simulink model "TV_lisb"  (R2024b)
settings: Solver=VariableStepAuto  StartTime=0.0  StopTime=10.0  RelTol=1e-3
PreLoadFcn:
  | run("TV_lisb_helper_file.m")
PostLoadFcn:
  | run("TV_lisb_helper_file.m")
InitFcn:
  | run("TV_lisb_helper_file.m")
StartFcn:
  | run("TV_lisb_helper_file.m")
StopFcn:
  | run("TV_lisb_helper_file.m")
model workspace: external: MATLAB File C:\Users\USER\Documents\MATLAB\NR\Git\TV_lisb_helper_file.m (data not in the file)
values from neighbouring files (symbols this model uses):
  C1 = 1.28    [TV_lisb_helper_file.m]
  C2 = 23.99    [TV_lisb_helper_file.m]
  C3 = 0.52    [TV_lisb_helper_file.m]
  C_roll = 0.01    [TV_lisb_helper_file.m]
  lf = 1.5    [TV_lisb_helper_file.m]
  lr = 1.5    [TV_lisb_helper_file.m]
  M = 300    [TV_lisb_helper_file.m]
  wr = 0.22    [TV_lisb_helper_file.m]
undefined symbols (not defined in the file or in its folder): g, tr
libraries: simulink x1
PreSaveFcn:
  | run("TV_lisb_helper_file.m")
PostSaveFcn:
  | run("TV_lisb_helper_file.m")
CloseFcn:
  | run("TV_lisb_helper_file.m")
PauseFcn:
  | run("TV_lisb_helper_file.m")
ContinueFcn:
  | run("TV_lisb_helper_file.m")
settings Model: Creator=USER  LastModifiedBy=USER

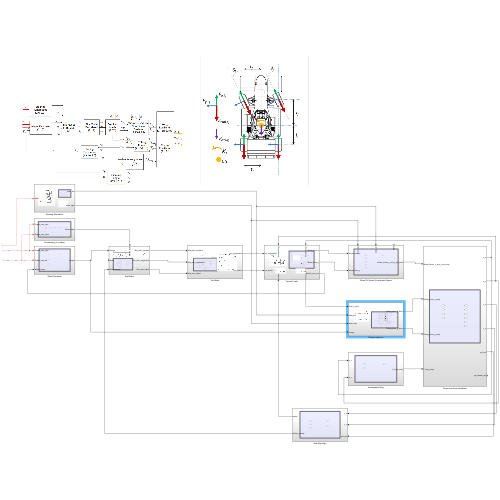
[thumbnail: Simulink's stored preview of the top-level diagram]
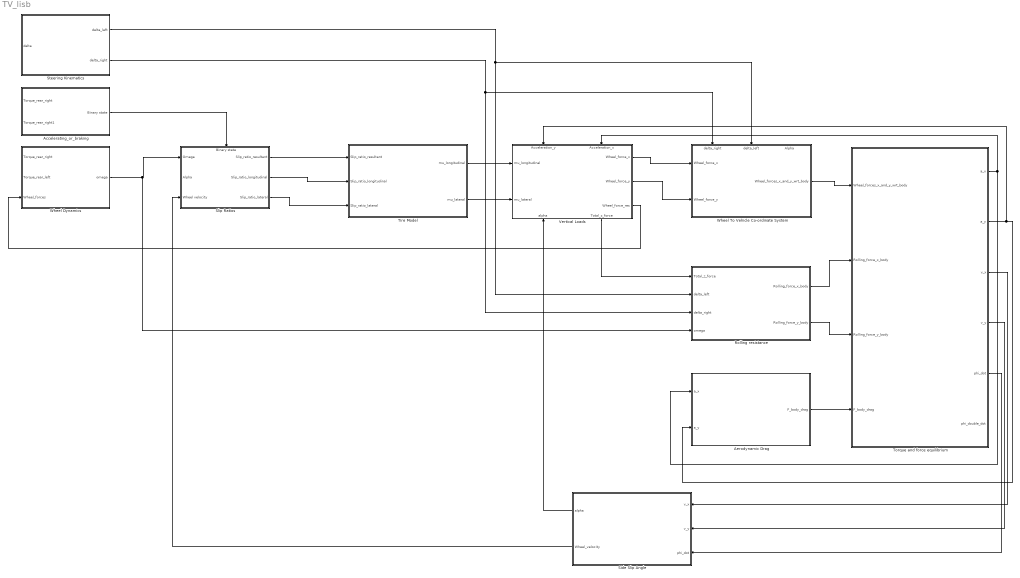
== system TV_lisb ==
  Accelerating_or_braking : Subsystem
  Aerodynamic Drag : Subsystem
  Rolling resistance : Subsystem
  Side Slip Angle : Subsystem
  Slip Ratios : Subsystem
      settings: PortSchema="{\"entries\":[{\"content\":{\"sides\":[{\"content\":{\"connectorIds\":[\"In1\",\"In2\",\"In3\"]},\"type\":\"ConnectorPlacement.EquallySpacedRectSide\",\"uuid\":\"f68f1183-9c60-479b-925c-3d4ffcaa1183\"},{\"content\":{\"connectorIds\":[\"Out1\",\"Out2\",\"Out3\"],\"side\":\"RIGHT\"},\"type\":\"ConnectorPlacement.EquallySpacedRectSide\",\"uuid\":\"3ccc78e5-55f6-4f64-bd15-35f9b9c5843d\"},{\"content\":{\"connectorIds\":[\"In4\"],\"side\":\"TOP\"},\"type\":\"ConnectorPlacement.EquallySpacedRectSide\",\"uuid\":\"873faff7-faeb-472b-bbf0-059c7e3a1cec\"}]},\"type\":\"ConnectorPlacement.EquallySpacedConnector\",\"uuid\":\"c1430164-14ee-465b-ad5a-b929bb7f1d2a\"}],\"packageUris\":[\"http://schema.mathworks.com/mf0/Connector/R2020b\"],\"version\":\"1.0\"}"
  Steering Kinematics : Subsystem
  Tire Model : Subsystem
  Torque and force equilibrium : Subsystem
  Vertical Loads : Subsystem
      settings: PortSchema="{\"entries\":[{\"content\":{\"sides\":[{\"content\":{\"connectorIds\":[\"In1\",\"In2\"]},\"type\":\"ConnectorPlacement.EquallySpacedRectSide\",\"uuid\":\"420474dd-77ae-41a3-b184-b8a376845dee\"},{\"content\":{\"connectorIds\":[\"Out1\",\"Out2\",\"Out3\"],\"side\":\"RIGHT\"},\"type\":\"ConnectorPlacement.EquallySpacedRectSide\",\"uuid\":\"e98bfd49-6816-4384-b726-feedfd108428\"},{\"content\":{\"connectorIds\":[\"In3\",\"In4\"],\"side\":\"TOP\"},\"type\":\"ConnectorPlacement.EquallySpacedRectSide\",\"uuid\":\"bc3c4692-54cb-49d4-bb5f-a504cda1efb8\"},{\"content\":{\"connectorIds\":[\"In5\",\"Out4\"],\"side\":\"BOTTOM\"},\"type\":\"ConnectorPlacement.EquallySpacedRectSide\",\"uuid\":\"ec39efe8-9589-4d25-8c83-c5c7b2f70cfd\"}]},\"type\":\"ConnectorPlacement.EquallySpacedConnector\",\"uuid\":\"6b01247e-c69a-46fe-b6d9-037bfd45934f\"}],\"packageUris\":[\"http://schema.mathworks.com/mf0/Connector/R2020b\"],\"version\":\"1.0\"}"
  Wheel Dynamics : Subsystem
  Wheel To Vehicle Co-ordinate System : Subsystem
      settings: PortSchema="{\"entries\":[{\"content\":{\"sides\":[{\"content\":{\"connectorIds\":[\"In1\",\"In2\"]},\"type\":\"ConnectorPlacement.EquallySpacedRectSide\",\"uuid\":\"1d639fc9-362c-4114-a9a5-2cccb0aa4f8f\"},{\"content\":{\"connectorIds\":[\"Out1\"],\"side\":\"RIGHT\"},\"type\":\"ConnectorPlacement.EquallySpacedRectSide\",\"uuid\":\"af7b8bc1-4639-4e57-ae25-0425d451201b\"},{\"content\":{\"connectorIds\":[\"In3\",\"In4\",\"In5\"],\"side\":\"TOP\"},\"type\":\"ConnectorPlacement.EquallySpacedRectSide\",\"uuid\":\"e7928f69-bff2-45cc-8c36-948ca369821c\"}]},\"type\":\"ConnectorPlacement.EquallySpacedConnector\",\"uuid\":\"c77d5f9f-6196-466d-893b-8bb143925d68\"}],\"packageUris\":[\"http://schema.mathworks.com/mf0/Connector/R2020b\"],\"version\":\"1.0\"}"
  wires:
  Slip Ratios/1(Slip_ratio_resultant) -> Tire Model/1(Slip_ratio_resultant)
  Wheel Dynamics/1(omega) -> Rolling resistance/4(omega), Slip Ratios/1(Omega)
  Vertical Loads/1(Wheel_force_x) -> Wheel To Vehicle Co-ordinate System/1(Wheel_force_x)
  Vertical Loads/2(Wheel_force_y) -> Wheel To Vehicle Co-ordinate System/2(Wheel_force_y)
  Steering Kinematics/2(delta_right) -> Rolling resistance/3(delta_right), Wheel To Vehicle Co-ordinate System/3(delta_right)
  Steering Kinematics/1(delta_left) -> Rolling resistance/2(delta_left), Wheel To Vehicle Co-ordinate System/4(delta_left)
  Wheel To Vehicle Co-ordinate System/1(Wheel_forces_x_and_y_wrt_body) -> Torque and force equilibrium/1(Wheel_forces_x_and_y_wrt_body)
  Vertical Loads/4(Total_z_force) -> Rolling resistance/1(Total_z_force)
  Rolling resistance/1(Rolling_force_x_body) -> Torque and force equilibrium/2(Rolling_force_x_body)
  Rolling resistance/2(Rolling_force_y_body) -> Torque and force equilibrium/3(Rolling_force_y_body)
  Aerodynamic Drag/1(F_body_drag) -> Torque and force equilibrium/4(F_body_drag)
  Torque and force equilibrium/1(a_x) -> Vertical Loads/4(Acceleration_x), Aerodynamic Drag/1(a_x)
  Torque and force equilibrium/2(a_y) -> Aerodynamic Drag/2(a_y), Vertical Loads/3(Acceleration_y)
  Vertical Loads/3(Wheel_force_res) -> Wheel Dynamics/3(Wheel_forces)
  Side Slip Angle/1(alpha) -> Vertical Loads/5(alpha)
  Side Slip Angle/2(Wheel_velocity) -> Slip Ratios/3(Wheel velocity)
  Torque and force equilibrium/3(v_x) -> Side Slip Angle/1(v_x)
  Torque and force equilibrium/4(v_y) -> Side Slip Angle/2(v_y)
  Torque and force equilibrium/5(phi_dot) -> Side Slip Angle/3(phi_dot)
  ? -> Accelerating_or_braking/1(Torque_rear_right), Wheel Dynamics/1(Torque_rear_right)
  ? -> Accelerating_or_braking/2(Torque_rear_right1), Wheel Dynamics/2(Torque_rear_left)
  Accelerating_or_braking/1(Binary state) -> Slip Ratios/4(Binary state)
  ? -> Steering Kinematics/1(delta)
  Slip Ratios/2(Slip_ratio_longitudinal) -> Tire Model/2(Slip_ratio_longitudinal)
  Slip Ratios/3(Slip_ratio_lateral) -> Tire Model/3(Slip_ratio_lateral)
  Tire Model/1(mu_longitudinal) -> Vertical Loads/1(mu_longitudinal)
  Tire Model/2(mu_lateral) -> Vertical Loads/2(mu_lateral)

== system TV_lisb/Accelerating_or_braking ==
  note: Gives 0 for braking, and 1 for accelerating
  Torque_rear_right : Inport
  Torque_rear_right1 : Inport  Port=2
  Add : Sum
  Compare To Zero : simulink/Logic and Bit Operations/Compare To Zero  relop=>=  OutDataTypeStr=uint8
  Derivative : Derivative
  Gain : Gain  Gain=0.5
  Binary state : Outport
  wires:
  Torque_rear_right/1 -> Add/1
  Torque_rear_right1/1 -> Add/2
  Add/1 -> Gain/1
  Gain/1 -> Derivative/1
  Derivative/1 -> Compare To Zero/1
  Compare To Zero/1 -> Binary state/1

== system TV_lisb/Aerodynamic Drag ==
  note: Aero calcs
  a_x : Inport
  a_y : Inport  Port=2
  F_body_drag : Outport

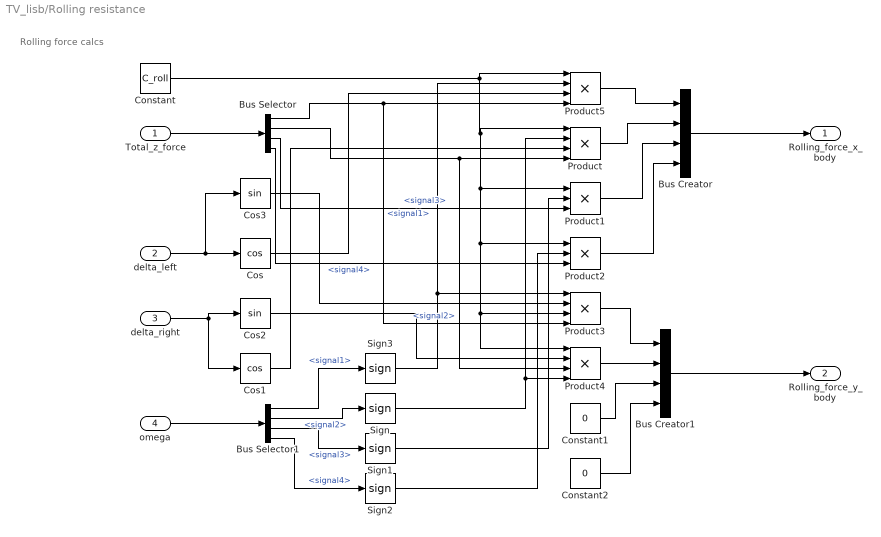
== system TV_lisb/Rolling resistance ==
  note: Rolling force calcs
  Total_z_force : Inport
  delta_left : Inport  Port=2
  delta_right : Inport  Port=3
  omega : Inport  Port=4
  Bus Creator : BusCreator  Inputs=4
  Bus Creator1 : BusCreator  Inputs=4
  Bus Selector : BusSelector  OutputSignals=signal1,signal2,signal3,signal4
  Bus Selector1 : BusSelector  OutputSignals=signal1,signal2,signal3,signal4
  Constant : Constant  Value=C_roll
  Constant1 : Constant  Value=0
  Constant2 : Constant  Value=0
  Cos : Trigonometry  Operator=cos
  Cos1 : Trigonometry  Operator=cos
  Cos2 : Trigonometry
  Cos3 : Trigonometry
  Product{,3..5} (4 alike) : Product  Inputs=4
  Product1 : Product  Inputs=3
  Product2 : Product  Inputs=3
  Sign{,1..3} (4 alike) : Signum
  Rolling_force_x_body : Outport
  Rolling_force_y_body : Outport  Port=2
  wires:
  Total_z_force/1 -> Bus Selector/1
  omega/1 -> Bus Selector1/1
  delta_left/1 -> Cos3/1, Cos/1
  delta_right/1 -> Cos2/1, Cos1/1
  Bus Selector1/1 -> Sign3/1  "<signal1>"
  Bus Selector1/2 -> Sign/1  "<signal2>"
  Bus Selector1/3 -> Sign1/1  "<signal3>"
  Bus Selector1/4 -> Sign2/1  "<signal4>"
  Constant/1 -> Product4/1, Product3/3, Product2/1, Product1/1, Product/1, Product5/1
  Bus Selector/1 -> Product3/4, Product5/4  "<signal1>"
  Sign3/1 -> Product3/1, Product5/2
  Cos/1 -> Product5/3
  Bus Selector/2 -> Product4/3, Product/4  "<signal2>"
  Sign/1 -> Product/2, Product4/4
  Cos1/1 -> Product/3
  Bus Selector/3 -> Product1/3  "<signal3>"
  Bus Selector/4 -> Product2/3  "<signal4>"
  Sign1/1 -> Product1/2
  Sign2/1 -> Product2/2
  Bus Creator/1 -> Rolling_force_x_body/1
  Product5/1 -> Bus Creator/1
  Product/1 -> Bus Creator/2
  Product1/1 -> Bus Creator/3
  Product2/1 -> Bus Creator/4
  Bus Creator1/1 -> Rolling_force_y_body/1
  Constant2/1 -> Bus Creator1/4
  Constant1/1 -> Bus Creator1/3
  Product4/1 -> Bus Creator1/2
  Product3/1 -> Bus Creator1/1
  Cos3/1 -> Product3/2
  Cos2/1 -> Product4/2

== system TV_lisb/Side Slip Angle ==
  note: Slip angle calcs
  v_x : Inport
  v_y : Inport  Port=2
  phi_dot : Inport  Port=3
  alpha : Outport
  Wheel_velocity : Outport  Port=2

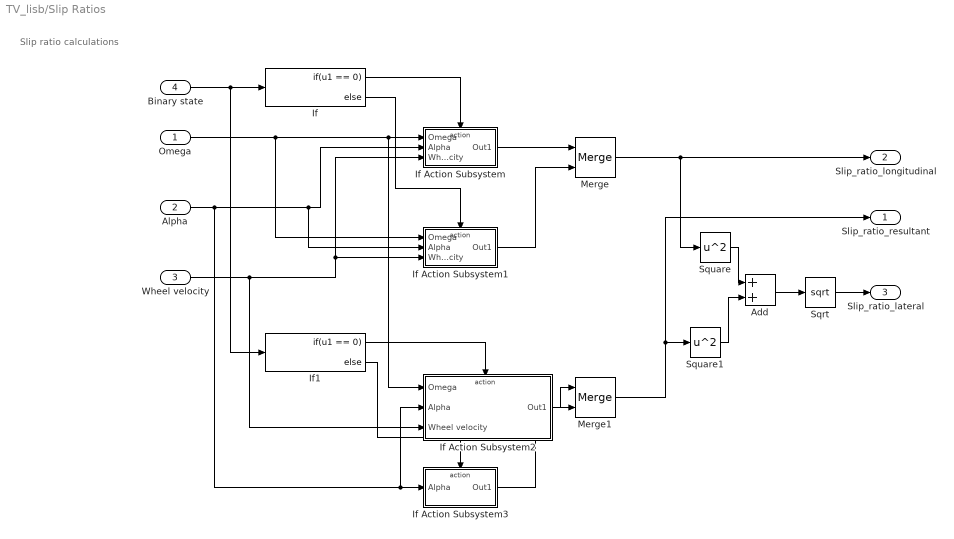
== system TV_lisb/Slip Ratios ==
  note: Slip ratio calculations
  Omega : Inport
  Alpha : Inport  Port=2
  Wheel velocity : Inport  Port=3
  Binary state : Inport  Port=4
  Add : Sum
  If : If  IfExpression=u1 == 0
  If Action Subsystem : Subsystem  TreatAsAtomicUnit=on
  If Action Subsystem1 : Subsystem  TreatAsAtomicUnit=on
  If Action Subsystem2 : Subsystem  TreatAsAtomicUnit=on
  If Action Subsystem3 : Subsystem  TreatAsAtomicUnit=on
  If1 : If  IfExpression=u1 == 0
  Merge : Merge
  Merge1 : Merge
  Sqrt : Sqrt
  Square : Math  Operator=square
  Square1 : Math  Operator=square
  Slip_ratio_resultant : Outport
  Slip_ratio_longitudinal : Outport  Port=2
  Slip_ratio_lateral : Outport  Port=3
  wires:
  Binary state/1 -> If/1, If1/1
  If/1 -> If Action Subsystem/Action
  If/2 -> If Action Subsystem1/Action
  Omega/1 -> If Action Subsystem2/1(Omega), If Action Subsystem/1(Omega), If Action Subsystem1/1(Omega)
  Alpha/1 -> If Action Subsystem1/2(Alpha), If Action Subsystem/2(Alpha), If Action Subsystem2/2(Alpha), If Action Subsystem3/1(Alpha)
  Wheel velocity/1 -> If Action Subsystem2/3(Wheel velocity), If Action Subsystem1/3(Wheel velocity), If Action Subsystem/3(Wheel velocity)
  If Action Subsystem/1(Out1) -> Merge/1
  If Action Subsystem1/1(Out1) -> Merge/2
  Merge/1 -> Square/1, Slip_ratio_longitudinal/1
  If Action Subsystem2/1(Out1) -> Merge1/1
  If Action Subsystem3/1(Out1) -> Merge1/2
  Merge1/1 -> Square1/1, Slip_ratio_resultant/1
  If1/1 -> If Action Subsystem2/Action
  If1/2 -> If Action Subsystem3/Action
  Sqrt/1 -> Slip_ratio_lateral/1
  Add/1 -> Sqrt/1
  Square/1 -> Add/1
  Square1/1 -> Add/2

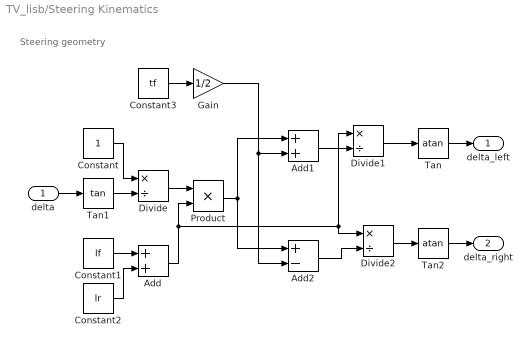
== system TV_lisb/Steering Kinematics ==
  note: Steering geometry
  delta : Inport
  Add : Sum
  Add1 : Sum
  Add2 : Sum  Inputs=+-
  Constant : Constant
  Constant1 : Constant  Value=lf
  Constant2 : Constant  Value=lr
  Constant3 : Constant  Value=tf
  Divide : Product  Inputs=*/
  Divide1 : Product  Inputs=*/
  Divide2 : Product  Inputs=*/
  Gain : Gain  Gain=1/2
  Product : Product
  Tan : Trigonometry  Operator=atan
  Tan1 : Trigonometry  Operator=tan
  Tan2 : Trigonometry  Operator=atan
  delta_left : Outport
  delta_right : Outport  Port=2
  wires:
  Tan/1 -> delta_left/1
  delta/1 -> Tan1/1
  Tan1/1 -> Divide/2
  Constant/1 -> Divide/1
  Constant1/1 -> Add/1
  Constant2/1 -> Add/2
  Divide/1 -> Product/1
  Add/1 -> Divide1/1, Divide2/1, Product/2
  Tan2/1 -> delta_right/1
  Constant3/1 -> Gain/1
  Gain/1 -> Add2/2, Add1/2
  Product/1 -> Add2/1, Add1/1
  Add1/1 -> Divide1/2
  Add2/1 -> Divide2/2
  Divide1/1 -> Tan/1
  Divide2/1 -> Tan2/1

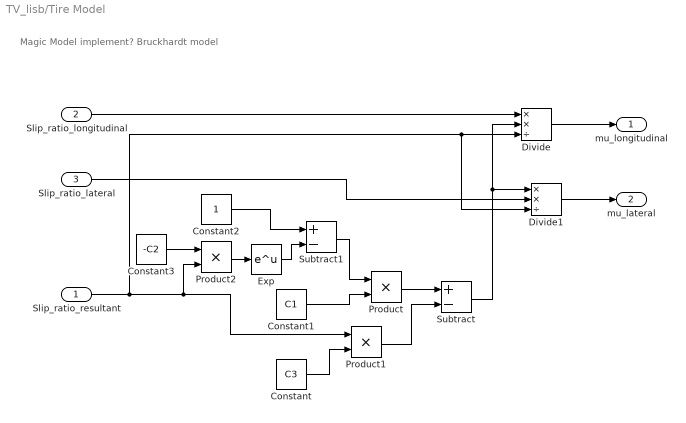
== system TV_lisb/Tire Model ==
  note: Magic Model implement?
      | Bruckhardt model
  Slip_ratio_resultant : Inport
  Slip_ratio_longitudinal : Inport  Port=2
  Slip_ratio_lateral : Inport  Port=3
  Constant : Constant  Value=C3
  Constant1 : Constant  Value=C1
  Constant2 : Constant
  Constant3 : Constant  Value=-C2
  Divide : Product  Inputs=**/
  Divide1 : Product  Inputs=**/
  Exp : Math
  Product : Product
  Product1 : Product
  Product2 : Product
  Subtract : Sum  Inputs=+-
  Subtract1 : Sum  Inputs=+-
  mu_longitudinal : Outport
  mu_lateral : Outport  Port=2
  wires:
  Product/1 -> Subtract/1
  Product1/1 -> Subtract/2
  Subtract/1 -> Divide/2, Divide1/1
  Slip_ratio_resultant/1 -> Divide1/3, Divide/3, Product2/2, Product1/1
  Constant/1 -> Product1/2
  Constant1/1 -> Product/2
  Subtract1/1 -> Product/1
  Constant2/1 -> Subtract1/1
  Constant3/1 -> Product2/1
  Exp/1 -> Subtract1/2
  Product2/1 -> Exp/1
  Divide/1 -> mu_longitudinal/1
  Slip_ratio_longitudinal/1 -> Divide/1
  Divide1/1 -> mu_lateral/1
  Slip_ratio_lateral/1 -> Divide1/2

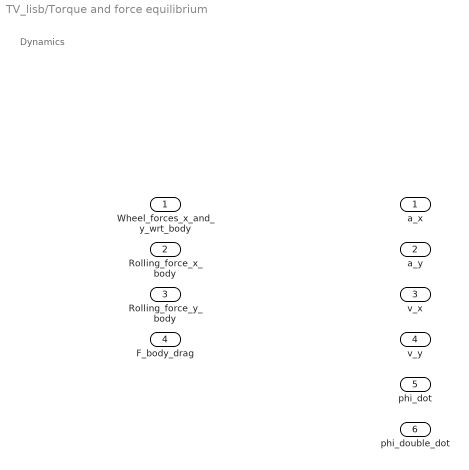
== system TV_lisb/Torque and force equilibrium ==
  note: Dynamics
  Wheel_forces_x_and_y_wrt_body : Inport
  Rolling_force_x_body : Inport  Port=2
  Rolling_force_y_body : Inport  Port=3
  F_body_drag : Inport  Port=4
  a_x : Outport
  a_y : Outport  Port=2
  v_x : Outport  Port=3
  v_y : Outport  Port=4
  phi_dot : Outport  Port=5
  phi_double_dot : Outport  Port=6

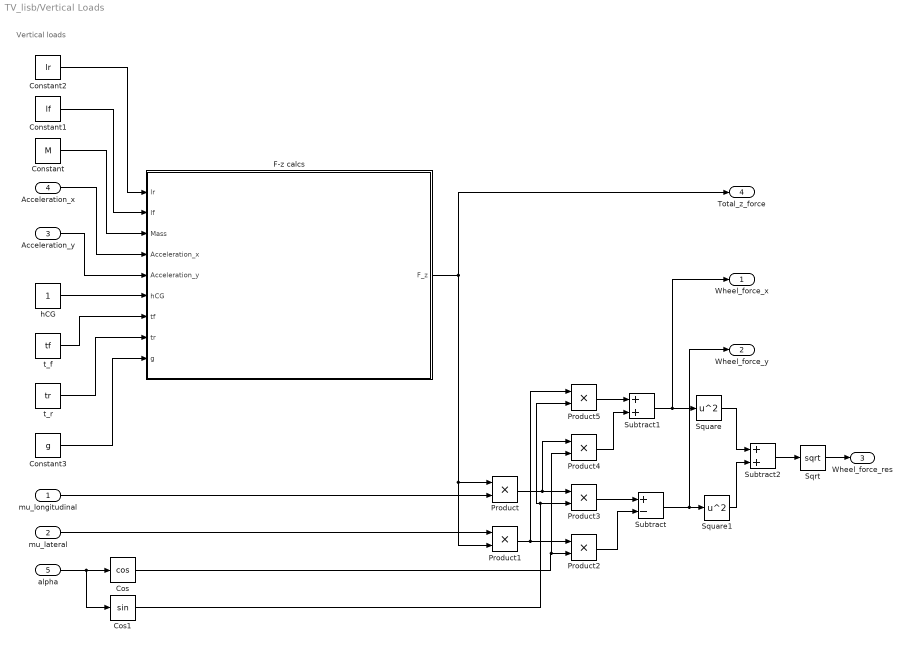
== system TV_lisb/Vertical Loads ==
  note: Vertical loads
  mu_longitudinal : Inport
  mu_lateral : Inport  Port=2
  Acceleration_y : Inport  Port=3
  Acceleration_x : Inport  Port=4
  alpha : Inport  Port=5
  Constant : Constant  Value=M
  Constant1 : Constant  Value=lf
  Constant2 : Constant  Value=lr
  Constant3 : Constant  Value=g
  Cos : Trigonometry  Operator=cos
  Cos1 : Trigonometry
  F-z calcs : Subsystem
  Product{,1..5} (6 alike) : Product
  Sqrt : Sqrt
  Square : Math  Operator=square
  Square1 : Math  Operator=square
  Subtract : Sum  Inputs=+-
  Subtract1 : Sum
  Subtract2 : Sum
  hCG : Constant
  t_f : Constant  Value=tf
  t_r : Constant  Value=tr
  Wheel_force_x : Outport
  Wheel_force_y : Outport  Port=2
  Wheel_force_res : Outport  Port=3
  Total_z_force : Outport  Port=4
  wires:
  Constant/1 -> F-z calcs/3(Mass)
  Constant2/1 -> F-z calcs/1(lr)
  Constant1/1 -> F-z calcs/2(lf)
  Acceleration_x/1 -> F-z calcs/4(Acceleration_x)
  Acceleration_y/1 -> F-z calcs/5(Acceleration_y)
  hCG/1 -> F-z calcs/6(hCG)
  t_f/1 -> F-z calcs/7(tf)
  Constant3/1 -> F-z calcs/9(g)
  t_r/1 -> F-z calcs/8(tr)
  F-z calcs/1(F_z) -> Product1/2, Product/1, Total_z_force/1
  mu_longitudinal/1 -> Product/2
  mu_lateral/1 -> Product1/1
  alpha/1 -> Cos1/1, Cos/1
  Cos/1 -> Product4/2, Product2/2
  Product1/1 -> Product5/1, Product2/1
  Product/1 -> Product4/1, Product3/1
  Cos1/1 -> Product5/2, Product3/2
  Product3/1 -> Subtract/1
  Product2/1 -> Subtract/2
  Subtract/1 -> Square1/1, Wheel_force_y/1
  Product5/1 -> Subtract1/1
  Product4/1 -> Subtract1/2
  Subtract1/1 -> Square/1, Wheel_force_x/1
  Subtract2/1 -> Sqrt/1
  Square1/1 -> Subtract2/2
  Square/1 -> Subtract2/1
  Sqrt/1 -> Wheel_force_res/1

== system TV_lisb/Wheel Dynamics ==
  note: Wheel Dynamics
  Torque_rear_right : Inport
  Torque_rear_left : Inport  Port=2
  Wheel_forces : Inport  Port=3
  omega : Outport

== system TV_lisb/Wheel To Vehicle Co-ordinate System ==
  note: Co-ordinate calculations
  Wheel_force_x : Inport
  Wheel_force_y : Inport  Port=2
  delta_right : Inport  Port=3
  delta_left : Inport  Port=4
  Alpha : Inport  Port=5
  Wheel_forces_x_and_y_wrt_body : Outport

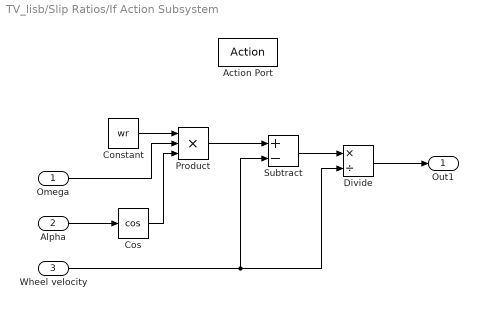
== system TV_lisb/Slip Ratios/If Action Subsystem ==
  Omega : Inport
  Alpha : Inport  Port=2
  Wheel velocity : Inport  Port=3
  Action Port : ActionPort  ActionPortLabel=if(u1 > 0)
  Constant : Constant  Value=wr
  Cos : Trigonometry  Operator=cos
  Divide : Product  Inputs=*/
  Product : Product  Inputs=3
  Subtract : Sum  Inputs=+-
  Out1 : Outport
  wires:
  Constant/1 -> Product/1
  Omega/1 -> Product/2
  Alpha/1 -> Cos/1
  Cos/1 -> Product/3
  Product/1 -> Subtract/1
  Wheel velocity/1 -> Divide/2, Subtract/2
  Subtract/1 -> Divide/1
  Divide/1 -> Out1/1

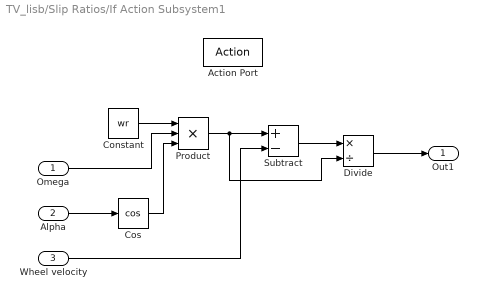
== system TV_lisb/Slip Ratios/If Action Subsystem1 ==
  Omega : Inport
  Alpha : Inport  Port=2
  Wheel velocity : Inport  Port=3
  Action Port : ActionPort  ActionPortLabel=else
  Constant : Constant  Value=wr
  Cos : Trigonometry  Operator=cos
  Divide : Product  Inputs=*/
  Product : Product  Inputs=3
  Subtract : Sum  Inputs=+-
  Out1 : Outport
  wires:
  Product/1 -> Divide/2, Subtract/1
  Subtract/1 -> Divide/1
  Alpha/1 -> Cos/1
  Cos/1 -> Product/3
  Omega/1 -> Product/2
  Constant/1 -> Product/1
  Divide/1 -> Out1/1
  Wheel velocity/1 -> Subtract/2

== system TV_lisb/Slip Ratios/If Action Subsystem2 ==
  Omega : Inport
  Alpha : Inport  Port=2
  Wheel velocity : Inport  Port=3
  Action Port : ActionPort  ActionPortLabel=if(u1 == 0)
  Constant : Constant  Value=wr
  Cos : Trigonometry
  Divide : Product  Inputs=*/
  Product : Product  Inputs=3
  Out1 : Outport
  wires:
  Constant/1 -> Product/1
  Omega/1 -> Product/2
  Alpha/1 -> Cos/1
  Cos/1 -> Product/3
  Wheel velocity/1 -> Divide/2
  Product/1 -> Divide/1
  Divide/1 -> Out1/1

== system TV_lisb/Slip Ratios/If Action Subsystem3 ==
  Alpha : Inport
  Action Port : ActionPort  ActionPortLabel=else
  Tan : Trigonometry  Operator=tan
  Out1 : Outport
  wires:
  Alpha/1 -> Tan/1
  Tan/1 -> Out1/1

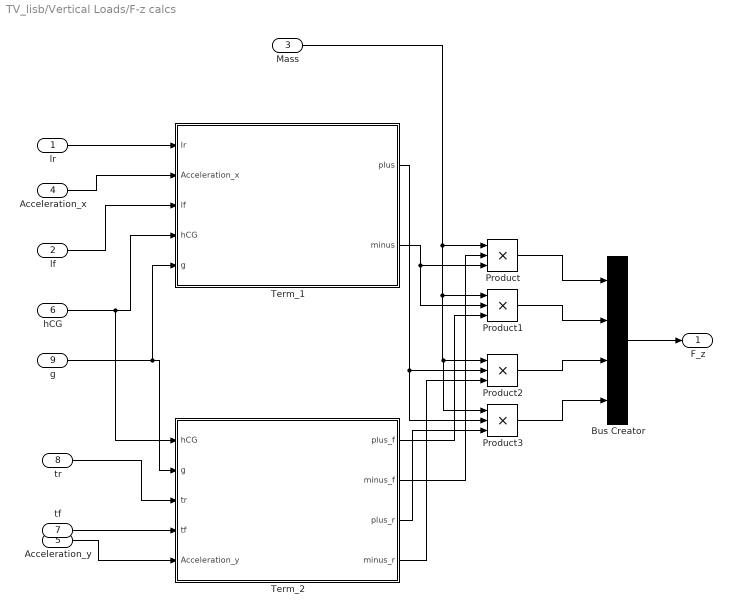
== system TV_lisb/Vertical Loads/F-z calcs ==
  lr : Inport
  lf : Inport  Port=2
  Mass : Inport  Port=3
  Acceleration_x : Inport  Port=4
  Acceleration_y : Inport  Port=5
  hCG : Inport  Port=6
  tf : Inport  Port=7
  tr : Inport  Port=8
  g : Inport  Port=9
  Bus Creator : BusCreator  Inputs=4
  Product{,1..3} (4 alike) : Product  Inputs=3
  Term_1 : Subsystem
  Term_2 : Subsystem
  F_z : Outport
  wires:
  lr/1 -> Term_1/1(lr)
  Acceleration_x/1 -> Term_1/2(Acceleration_x)
  lf/1 -> Term_1/3(lf)
  hCG/1 -> Term_2/1(hCG), Term_1/4(hCG)
  g/1 -> Term_2/2(g), Term_1/5(g)
  Acceleration_y/1 -> Term_2/5(Acceleration_y)
  tf/1 -> Term_2/4(tf)
  tr/1 -> Term_2/3(tr)
  Product/1 -> Bus Creator/1
  Product1/1 -> Bus Creator/2
  Product2/1 -> Bus Creator/3
  Product3/1 -> Bus Creator/4
  Mass/1 -> Product3/1, Product2/1, Product1/1, Product/1
  Term_1/2(minus) -> Product1/2, Product/3
  Term_2/2(minus_f) -> Product/2
  Term_2/1(plus_f) -> Product1/3
  Term_1/1(plus) -> Product3/2, Product2/2
  Term_2/4(minus_r) -> Product2/3
  Term_2/3(plus_r) -> Product3/3
  Bus Creator/1 -> F_z/1

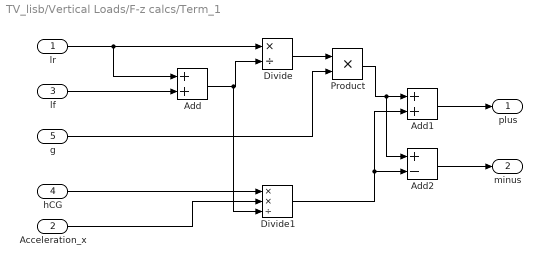
== system TV_lisb/Vertical Loads/F-z calcs/Term_1 ==
  lr : Inport
  Acceleration_x : Inport  Port=2
  lf : Inport  Port=3
  hCG : Inport  Port=4
  g : Inport  Port=5
  Add : Sum
  Add1 : Sum
  Add2 : Sum  Inputs=+-
  Divide : Product  Inputs=*/
  Divide1 : Product  Inputs=**/
  Product : Product
  plus : Outport
  minus : Outport  Port=2
  wires:
  lr/1 -> Add/1, Divide/1
  lf/1 -> Add/2
  Add/1 -> Divide1/3, Divide/2
  Divide/1 -> Product/1
  g/1 -> Product/2
  Product/1 -> Add2/1, Add1/1
  hCG/1 -> Divide1/1
  Acceleration_x/1 -> Divide1/2
  Divide1/1 -> Add2/2, Add1/2
  Add1/1 -> plus/1
  Add2/1 -> minus/1

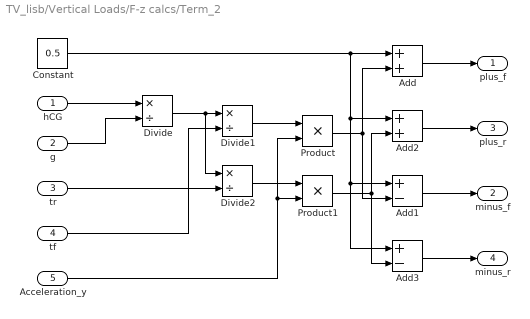
== system TV_lisb/Vertical Loads/F-z calcs/Term_2 ==
  hCG : Inport
  g : Inport  Port=2
  tr : Inport  Port=3
  tf : Inport  Port=4
  Acceleration_y : Inport  Port=5
  Add : Sum
  Add1 : Sum  Inputs=+-
  Add2 : Sum
  Add3 : Sum  Inputs=+-
  Constant : Constant  Value=0.5
  Divide : Product  Inputs=*/
  Divide1 : Product  Inputs=*/
  Divide2 : Product  Inputs=*/
  Product : Product
  Product1 : Product
  plus_f : Outport
  minus_f : Outport  Port=2
  plus_r : Outport  Port=3
  minus_r : Outport  Port=4
  wires:
  Add1/1 -> minus_f/1
  Add/1 -> plus_f/1
  hCG/1 -> Divide/1
  Add2/1 -> plus_r/1
  Add3/1 -> minus_r/1
  g/1 -> Divide/2
  Divide/1 -> Divide2/1, Divide1/1
  tf/1 -> Divide1/2
  Divide1/1 -> Product/1
  Acceleration_y/1 -> Product1/2, Product/2
  Product/1 -> Add/2, Add1/2
  Constant/1 -> Add3/1, Add1/1, Add2/1, Add/1
  tr/1 -> Divide2/2
  Divide2/1 -> Product1/1
  Product1/1 -> Add3/2, Add2/2
